simulink model "TESTENV_Task"  (R2020a)
settings: Solver=FixedStepAuto  StartTime=0.0  StopTime=4500  RelTol=1e-3
undefined symbols (not defined in the file or in its folder): airspeed1, ENUM_FlightTaskMode, ENUM_SensorHealthStatus, ENUM_SystemHealthStatus, FlightPerfParam_V10, FlightPerfParam_V1000, PlaneMode, radar1, SensorStatus, SystemHealthStatus, TaskParam_V10, TaskParam_V1000, windHeading_rad, windSpeed_ms
settings Model: PauseTimes=[500,868]  PacingRate=6  Creator=sl  LastModifiedBy=Administrator
settings DebuggingCC: InheritedTsInSrcMsg=none  ArithmeticOperatorsInVariantConditions=warning
settings ModelReferenceCC: PropagateVarSize=During execution
settings SFSimCC: CustomCodeUndefinedFunction=UseInterfaceOnly

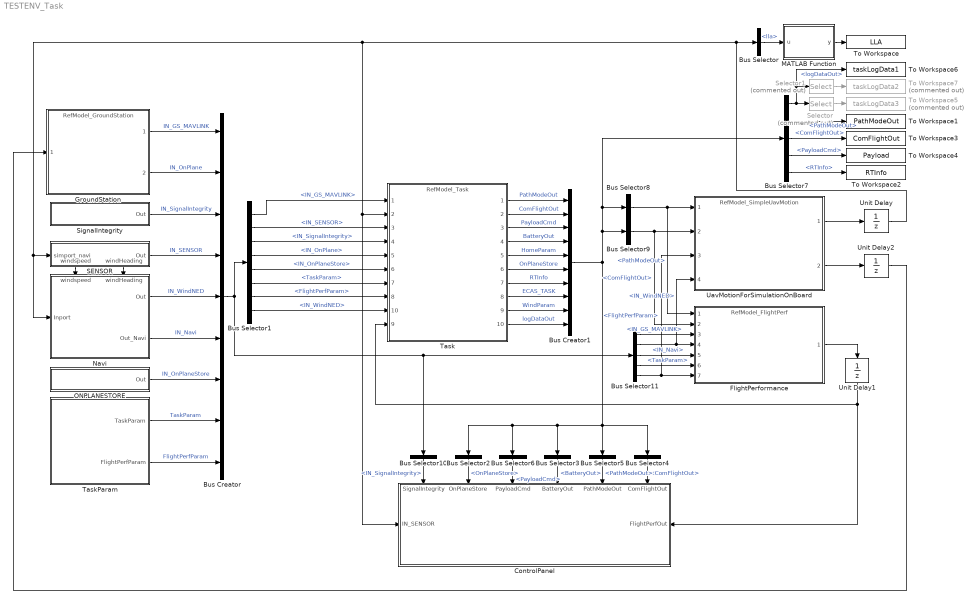
== system TESTENV_Task ==
  Bus Creator : BusCreator  Inputs=9
  Bus Creator1 : BusCreator  Inputs=10
  Bus Selector : BusSelector  OutputSignals=lla
  Bus Selector1 : BusSelector  OutputSignals=IN_GS_MAVLINK,IN_SENSOR,IN_SignalIntegrity,IN_OnPlane,IN_OnPlaneStore,TaskParam,FlightPerfParam,IN_WindNED
  Bus Selector10 : BusSelector  OutputSignals=IN_SignalIntegrity
  Bus Selector11 : BusSelector  OutputSignals=IN_GS_MAVLINK,IN_WindNED,IN_Navi,TaskParam,FlightPerfParam
  Bus Selector2 : BusSelector  OutputSignals=OnPlaneStore
  Bus Selector3 : BusSelector  OutputSignals=BatteryOut
  Bus Selector4 : BusSelector  OutputSignals=ComFlightOut
  Bus Selector5 : BusSelector  OutputSignals=PathModeOut
  Bus Selector6 : BusSelector  OutputSignals=PayloadCmd
  Bus Selector7 : BusSelector  OutputSignals=logDataOut,PathModeOut,ComFlightOut,PayloadCmd,RTInfo
  Bus Selector8 : BusSelector  OutputSignals=PathModeOut
  Bus Selector9 : BusSelector  OutputSignals=ComFlightOut
  ControlPanel : Subsystem
      settings: PortSchema="{\"entries\":[{\"content\":{\"sides\":[{\"content\":{\"connectorIds\":[]},\"type\":\"ConnectorPlacement.EquallySpacedRectSide\",\"uuid\":\"28eb3c17-6733-4c9d-9d3b-b06e91bad00c\"},{\"content\":{\"connectorIds\":[\"In3\",\"In4\",\"In5\",\"In6\",\"In7\",\"In8\"],\"side\":\"RIGHT\"},\"type\":\"ConnectorPlacement.EquallySpacedRectSide\",\"uuid\":\"44e37a17-9aaf-4985-a14b-a4ae4b690f0b\"},{\"content\":{\"connectorIds\":[\"In1\"],\"side\":\"TOP\"},\"type\":\"ConnectorPlacement.EquallySpacedRectSide\",\"uuid\":\"dc63a870-4d25-41e6-babc-24267acffaf6\"},{\"content\":{\"connectorIds\":[\"In2\"],\"side\":\"BOTTOM\"},\"type\":\"ConnectorPlacement.EquallySpacedRectSide\",\"uuid\":\"de4ecddf-9d24-4ca5-8235-aab9efd95b3c\"}]},\"type\":\"ConnectorPlacement.EquallySpacedConnector\",\"uuid\":\"a23d6a61-f1f8-4715-9225-859bb8c68d23\"}],\"packageUris\":[\"http://schema.mathworks.com/mf0/Connector/19700101\"],\"version\":\"1.0\"}"
  FlightPerformance : ModelReference  ModelNameDialog=RefModel_FlightPerf.slx  SimulationMode=Normal  CachedPortDiscreteRates=[0.04]  ModelReferenceVersion=1.3545
  GroundStation : ModelReference  ModelNameDialog=RefModel_GroundStation.slx  SimulationMode=Normal  CachedPortDiscreteRates=[0.04]  ModelReferenceVersion=1.3846
  MATLAB Function : MATLAB Function  TreatAsAtomicUnit=on
  Navi : Subsystem
      settings: PortSchema="{\"entries\":[{\"content\":{\"sides\":[{\"content\":{\"connectorIds\":[\"In1\"]},\"type\":\"ConnectorPlacement.EquallySpacedRectSide\",\"uuid\":\"f65589f5-bebe-42f0-87a0-22889f9d8cf8\"},{\"content\":{\"connectorIds\":[\"Out1\",\"Out2\"],\"side\":\"RIGHT\"},\"type\":\"ConnectorPlacement.EquallySpacedRectSide\",\"uuid\":\"9d118f62-a4fa-485f-8fb7-3972b29fb71e\"},{\"content\":{\"connectorIds\":[\"In2\",\"In3\"],\"side\":\"TOP\"},\"type\":\"ConnectorPlacement.EquallySpacedRectSide\",\"uuid\":\"31b3786a-ad94-4275-bb9f-8feeb00b35dc\"}]},\"type\":\"ConnectorPlacement.EquallySpacedConnector\",\"uuid\":\"aa2c1c65-c057-4fb8-aaff-4f4272248123\"}],\"packageUris\":[\"http://schema.mathworks.com/mf0/Connector/19700101\"],\"version\":\"1.0\"}"
  ONPLANESTORE : Subsystem
  SENSOR : Subsystem
      settings: PortSchema="{\"entries\":[{\"content\":{\"sides\":[{\"content\":{\"connectorIds\":[\"In1\"]},\"type\":\"ConnectorPlacement.EquallySpacedRectSide\",\"uuid\":\"ba991dc2-7a34-4bf6-a888-7f4af2e50d12\"},{\"content\":{\"connectorIds\":[\"Out1\"],\"side\":\"RIGHT\"},\"type\":\"ConnectorPlacement.EquallySpacedRectSide\",\"uuid\":\"c7226504-ba61-436f-baed-66203ae29e34\"},{\"content\":{\"connectorIds\":[],\"side\":\"TOP\"},\"type\":\"ConnectorPlacement.EquallySpacedRectSide\",\"uuid\":\"1861e618-12e2-4f65-bbab-d347bc046ba7\"},{\"content\":{\"connectorIds\":[\"Out2\",\"Out3\"],\"side\":\"BOTTOM\"},\"type\":\"ConnectorPlacement.EquallySpacedRectSide\",\"uuid\":\"711a3230-d97b-4007-957d-7ac810c9eb75\"}]},\"type\":\"ConnectorPlacement.EquallySpacedConnector\",\"uuid\":\"48c07c27-922c-4e4d-aad7-64a2a545d2e4\"}],\"packageUris\":[\"http://schema.mathworks.com/mf0/Connector/19700101\"],\"version\":\"1.0\"}"
  Selector : Selector  Commented=on  InputPortWidth=3  IndexOptions=Index vector (dialog)  Indices=3  OutputSizes=1
  Selector1 : Selector  Commented=on  InputPortWidth=3  IndexOptions=Index vector (dialog)  Indices=2  OutputSizes=1
  SignalIntegrity : Subsystem
  Task : ModelReference  ModelNameDialog=RefModel_Task.slx  SimulationMode=Normal  CachedPortDiscreteRates=[0.036]  ModelReferenceVersion=1.6002
      settings: PortSchema="{\"entries\":[{\"content\":{\"sides\":[{\"content\":{\"connectorIds\":[\"In1\",\"In2\",\"In3\",\"In4\",\"In5\",\"In6\",\"In7\",\"In8\",\"In10\",\"In9\"]},\"type\":\"ConnectorPlacement.EquallySpacedRectSide\",\"uuid\":\"d9fd24e3-43bd-49c5-a4e1-6245eb51949c\"},{\"content\":{\"connectorIds\":[\"Out1\",\"Out2\",\"Out3\",\"Out4\",\"Out5\",\"Out6\",\"Out7\",\"Out8\",\"Out9\",\"Out10\"],\"side\":\"RIGHT\"},\"type\":\"ConnectorPlacement.EquallySpacedRectSide\",\"uuid\":\"bf33909e-0e0f-4f0f-a250-56f1d45be6e7\"},{\"content\":{\"connectorIds\":[],\"side\":\"TOP\"},\"type\":\"ConnectorPlacement.EquallySpacedRectSide\",\"uuid\":\"77fc1f2c-3bac-4439-b1c1-53d076175420\"}]},\"type\":\"ConnectorPlacement.EquallySpacedConnector\",\"uuid\":\"17e9d58e-9274-43dc-be21-5439798aa13e\"}],\"packageUris\":[\"http://schema.mathworks.com/mf0/Connector/19700101\"],\"version\":\"1.0\"}"
  TaskParam : Subsystem
  To Workspace : ToWorkspace  VariableName=LLA  SaveFormat=Timeseries  SampleTime=-1
  To Workspace1 : ToWorkspace  VariableName=PathModeOut  SaveFormat=Timeseries  SampleTime=-1
  To Workspace2 : ToWorkspace  VariableName=RTInfo  SaveFormat=Timeseries  SampleTime=-1
  To Workspace3 : ToWorkspace  VariableName=ComFlightOut  SaveFormat=Timeseries  SampleTime=-1
  To Workspace4 : ToWorkspace  VariableName=Payload  SaveFormat=Timeseries  SampleTime=-1
  To Workspace5 : ToWorkspace  Commented=on  VariableName=taskLogData3  SaveFormat=Timeseries  SampleTime=-1
  To Workspace6 : ToWorkspace  VariableName=taskLogData1  SaveFormat=Timeseries  SampleTime=-1
  To Workspace7 : ToWorkspace  Commented=on  VariableName=taskLogData2  SaveFormat=Timeseries  SampleTime=-1
  UavMotionForSimulationOnBoard : ModelReference  ModelNameDialog=RefModel_SimpleUavMotion.slx  SimulationMode=Normal  CachedPortDiscreteRates=[0.04]  ModelReferenceVersion=1.1044
  Unit Delay : UnitDelay  SampleTime=-1  HasFrameUpgradeWarning=on
  Unit Delay1 : UnitDelay  SampleTime=-1  HasFrameUpgradeWarning=on
  Unit Delay2 : UnitDelay  SampleTime=-1  HasFrameUpgradeWarning=on
  wires:
  GroundStation/1 -> Bus Creator/1  "IN_GS_MAVLINK"
  SignalIntegrity/1(Out) -> Bus Creator/3  "IN_SignalIntegrity"
  GroundStation/2 -> Bus Creator/2  "IN_OnPlane"
  UavMotionForSimulationOnBoard/1 -> Unit Delay/1
  Unit Delay/1 -> ControlPanel/1(IN_SENSOR), Task/2, Navi/1(Inport), SENSOR/1(simport_navi), Bus Selector/1
  Bus Selector/1 -> MATLAB Function/1(u)  "<lla>"
  MATLAB Function/1(y) -> To Workspace/1
  SENSOR/1(Out) -> Bus Creator/4  "IN_SENSOR"
  ONPLANESTORE/1(Out) -> Bus Creator/7  "IN_OnPlaneStore"
  FlightPerformance/1 -> Unit Delay1/1
  Bus Selector1/6 -> Task/7  "<TaskParam>"
  Bus Creator/1 -> Bus Selector1/1, Bus Selector10/1, Bus Selector11/1
  Bus Selector1/1 -> Task/1  "<IN_GS_MAVLINK>"
  Bus Selector1/3 -> Task/4  "<IN_SignalIntegrity>"
  Bus Selector1/2 -> Task/3  "<IN_SENSOR>"
  Bus Selector1/4 -> Task/5  "<IN_OnPlane>"
  Bus Selector1/5 -> Task/6  "<IN_OnPlaneStore>"
  Task/1 -> Bus Creator1/1  "PathModeOut"
  Task/2 -> Bus Creator1/2  "ComFlightOut"
  Task/3 -> Bus Creator1/3  "PayloadCmd"
  Task/4 -> Bus Creator1/4  "BatteryOut"
  Task/5 -> Bus Creator1/5  "HomeParam"
  Task/6 -> Bus Creator1/6  "OnPlaneStore"
  Task/7 -> Bus Creator1/7  "RTInfo"
  Task/8 -> Bus Creator1/8  "ECAS_TASK"
  Task/9 -> Bus Creator1/9  "WindParam"
  Bus Selector2/1 -> ControlPanel/4(OnPlaneStore)  "<OnPlaneStore>"
  Bus Selector3/1 -> ControlPanel/6(BatteryOut)  "<BatteryOut>"
  Bus Selector4/1 -> ControlPanel/8(ComFlightOut)  "<ComFlightOut>"
  Bus Selector5/1 -> ControlPanel/7(PathModeOut)  "<PathModeOut>"
  Bus Selector6/1 -> ControlPanel/5(PayloadCmd)  "<PayloadCmd>"
  Bus Creator1/1 -> Bus Selector9/1, Bus Selector8/1, Bus Selector7/1, Bus Selector3/1, Bus Selector6/1, Bus Selector2/1, Bus Selector5/1, Bus Selector4/1
  Bus Selector7/5 -> To Workspace2/1  "<RTInfo>"
  Bus Selector7/2 -> To Workspace1/1  "<PathModeOut>"
  Bus Selector7/3 -> To Workspace3/1  "<ComFlightOut>"
  Bus Selector7/4 -> To Workspace4/1  "<PayloadCmd>"
  Bus Selector8/1 -> FlightPerformance/1, UavMotionForSimulationOnBoard/1  "<PathModeOut>"
  Bus Selector9/1 -> FlightPerformance/2, UavMotionForSimulationOnBoard/2  "<ComFlightOut>"
  Bus Selector10/1 -> ControlPanel/3(SignalIntegrity)  "<IN_SignalIntegrity>"
  Bus Selector11/1 -> FlightPerformance/3  "<IN_GS_MAVLINK>"
  Unit Delay1/1 -> Task/9, ControlPanel/2(FlightPerfOut)
  Navi/1(Out) -> Bus Creator/5  "IN_WindNED"
  SENSOR/2(windspeed) -> Navi/2(windspeed)
  Bus Selector1/8 -> Task/10  "<IN_WindNED>"
  Bus Selector11/2 -> FlightPerformance/4, UavMotionForSimulationOnBoard/4  "<IN_WindNED>"
  UavMotionForSimulationOnBoard/2 -> Unit Delay2/1
  Unit Delay2/1 -> GroundStation/1
  Task/10 -> Bus Creator1/10  "logDataOut"
  Bus Selector7/1 -> To Workspace6/1, Selector1/1, Selector/1  "<logDataOut>"
  Selector/1 -> To Workspace5/1
  Selector1/1 -> To Workspace7/1
  SENSOR/3(windHeading) -> Navi/3(windHeading)
  TaskParam/1(TaskParam) -> Bus Creator/8  "TaskParam"
  Navi/2(Out_Navi) -> Bus Creator/6  "IN_Navi"
  Bus Selector11/3 -> FlightPerformance/5  "<IN_Navi>"
  Bus Selector11/4 -> FlightPerformance/6  "<TaskParam>"
  TaskParam/2(FlightPerfParam) -> Bus Creator/9  "FlightPerfParam"
  Bus Selector1/7 -> Task/8  "<FlightPerfParam>"
  Bus Selector11/5 -> FlightPerformance/7, UavMotionForSimulationOnBoard/3  "<FlightPerfParam>"

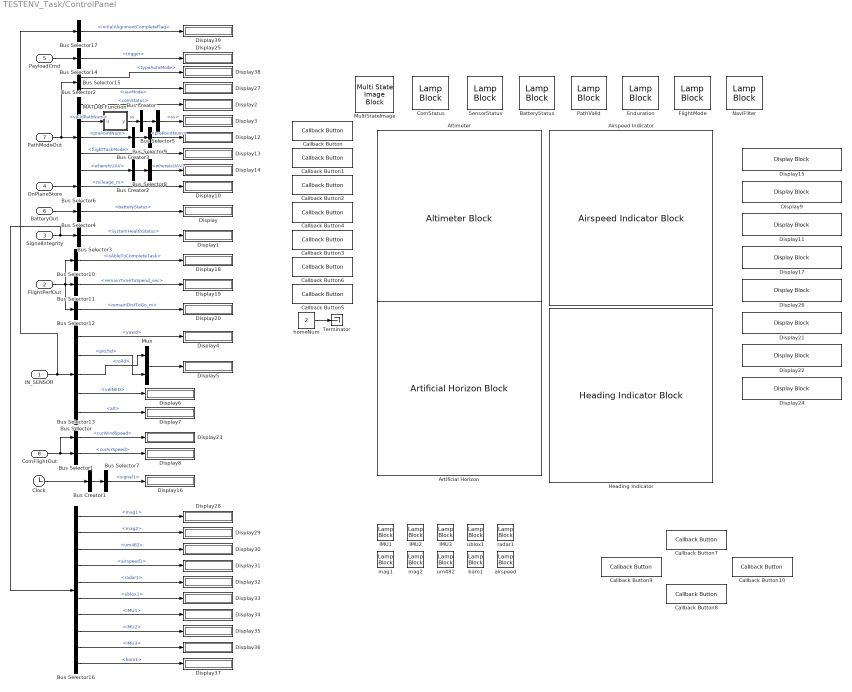
== system TESTENV_Task/ControlPanel ==
  IN_SENSOR : Inport
  FlightPerfOut : Inport  Port=2
  SignalIntegrity : Inport  Port=3
  OnPlaneStore : Inport  Port=4
  PayloadCmd : Inport  Port=5
  BatteryOut : Inport  Port=6
  PathModeOut : Inport  Port=7
  ComFlightOut : Inport  Port=8
  Airspeed Indicator : AirspeedIndicatorBlock  ScaleMin=-10  ScaleMax=50
  Altimeter : AltimeterBlock
  Artificial Horizon : ArtificialHorizonBlock
  BatteryStatus : LampBlock
  Bus Creator{,1..3} (4 alike) : BusCreator  Inputs=1
  Bus Selector : BusSelector  OutputSignals=yawd,pitchd,rolld,velNED,alt
  Bus Selector1 : BusSelector  OutputSignals=curAirSpeed
  Bus Selector10 : BusSelector  OutputSignals=isAbleToCompleteTask
  Bus Selector11 : BusSelector  OutputSignals=remainTimeToSpend_sec
  Bus Selector12 : BusSelector  OutputSignals=remainDistToGo_m
  Bus Selector13 : BusSelector  OutputSignals=curWindSpeed
  Bus Selector14 : BusSelector  OutputSignals=CAMERA.trigger
  Bus Selector15 : BusSelector  OutputSignals=typeAutoMode,uavMode
  Bus Selector16 : BusSelector  OutputSignals=SensorStatus.mag1,SensorStatus.mag2,SensorStatus.um482,SensorStatus.airspeed1,SensorStatus.radar1,SensorStatus.ublox1,SensorStatus.IMU1,SensorStatus.IMU2,SensorStatus.IMU3,SensorStatus.baro1
  Bus Selector17 : BusSelector  OutputSignals=initialAlignmentCompleteFlag
  Bus Selector2 : BusSelector  OutputSignals=comStatus,validPathNum,prePointNum,flightTaskMode,whereIsUAV
  Bus Selector3 : BusSelector  OutputSignals=SystemHealthStatus
  Bus Selector4 : BusSelector  OutputSignals=batteryStatus
  Bus Selector5 : BusSelector  OutputSignals=ss
  Bus Selector6 : BusSelector  OutputSignals=mileage_m
  Bus Selector7 : BusSelector  OutputSignals=signal1
  Bus Selector8 : BusSelector  OutputSignals=whereIsUAV
  Bus Selector9 : BusSelector  OutputSignals=prePointNum
  Callback Button : CallbackButton  ButtonText=起飞
      settings: ClickFcn=|
      | set_param('RefModel_GroundStation/GSButton','value','5')
      | tmpVal = get_param('RefModel_GroundStation/mav_command_long_recvflag','value');
      | tmpVal = str2double(tmpVal);
      | set_param('RefModel_GroundStation/mav_command_long_recvflag','value',num2str(tmpVal+1))
  Callback Button1 : CallbackButton  ButtonText=开始任务
      settings: ClickFcn=|
      | set_param('RefModel_GroundStation/GSButton','value','4')
      | tmpVal = get_param('RefModel_GroundStation/mav_command_long_recvflag','value');
      | tmpVal = str2double(tmpVal);
      | set_param('RefModel_GroundStation/mav_command_long_recvflag','value',num2str(tmpVal+1))
  Callback Button10 : CallbackButton  ButtonText=右+5
      settings: ClickFcn=|
      | tmpVal = get_param('RefModel_GroundStation/mavlink_msg_arrowkey/nRight','value');
      | tmpVal = str2double(tmpVal);
      | set_param('RefModel_GroundStation/mavlink_msg_arrowkey/nRight','value',num2str(tmpVal+5))
  Callback Button2 : CallbackButton  ButtonText=暂停
      settings: ClickFcn=|
      | set_param('RefModel_GroundStation/GSButton','value','3')
      | tmpVal = get_param('RefModel_GroundStation/mav_command_long_recvflag','value');
      | tmpVal = str2double(tmpVal);
      | set_param('RefModel_GroundStation/mav_command_long_recvflag','value',num2str(tmpVal+1))
  Callback Button3 : CallbackButton  ButtonText=返航
      settings: ClickFcn=|
      | set_param('RefModel_GroundStation/GSButton','value','2')
      | tmpVal = get_param('RefModel_GroundStation/mav_command_long_recvflag','value');
      | tmpVal = str2double(tmpVal);
      | set_param('RefModel_GroundStation/mav_command_long_recvflag','value',num2str(tmpVal+1))
  Callback Button4 : CallbackButton  ButtonText=固定翼转旋翼
      settings: ClickFcn=|
      | set_param('RefModel_GroundStation/GSButton','value','14')
      | tmpVal = get_param('RefModel_GroundStation/mav_command_long_recvflag','value');
      | tmpVal = str2double(tmpVal);
      | set_param('RefModel_GroundStation/mav_command_long_recvflag','value',num2str(tmpVal+1))
  Callback Button5 : CallbackButton  ButtonText=修改HOME点
      settings: ClickFcn=|
      | tmpVal = get_param('TESTENV_Task/ControlPanel/homeNum','value');
      | tmpVal = str2double(tmpVal);
      | if tmpVal > 4
      |     tmpVal = 4;
      | elseif tmpVal < 1
      |     tmpVal = 1;
      | end
      | set_param('RefModel_GroundStation/PathPoints/HomeNumSel','value',num2str(tmpVal))
  Callback Button6 : CallbackButton  ButtonText=一键降落
      settings: ClickFcn=|
      | set_param('RefModel_GroundStation/GSButton','value','7')
      | tmpVal = get_param('RefModel_GroundStation/mav_command_long_recvflag','value');
      | tmpVal = str2double(tmpVal);
      | set_param('RefModel_GroundStation/mav_command_long_recvflag','value',num2str(tmpVal+1))
  Callback Button7 : CallbackButton  ButtonText=前+5
      settings: ClickFcn=|
      | tmpVal = get_param('RefModel_GroundStation/mavlink_msg_arrowkey/nFront','value');
      | tmpVal = str2double(tmpVal);
      | set_param('RefModel_GroundStation/mavlink_msg_arrowkey/nFront','value',num2str(tmpVal+5))
  Callback Button8 : CallbackButton  ButtonText=后+5
      settings: ClickFcn=|
      | tmpVal = get_param('RefModel_GroundStation/mavlink_msg_arrowkey/nBack','value');
      | tmpVal = str2double(tmpVal);
      | set_param('RefModel_GroundStation/mavlink_msg_arrowkey/nBack','value',num2str(tmpVal+5))
  Callback Button9 : CallbackButton  ButtonText=左+5
      settings: ClickFcn=|
      | tmpVal = get_param('RefModel_GroundStation/mavlink_msg_arrowkey/nLeft','value');
      | tmpVal = str2double(tmpVal);
      | set_param('RefModel_GroundStation/mavlink_msg_arrowkey/nLeft','value',num2str(tmpVal+5))
  Clock : Clock
  ComStatus : LampBlock
  Display{,1..8,10,12..14,16,18..20,23,25,27..39} (32 alike) : Display
  Display11 : DisplayBlock  Format=Custom  Transparency=1  FormatString=时间 %.1f [sec]
  Display15 : DisplayBlock  Format=Custom  Transparency=1  FormatString=%s
  Display17 : DisplayBlock  Format=Custom  Transparency=1  FormatString=航点 %d
  Display21 : DisplayBlock  Format=Custom  Transparency=1  FormatString=剩余时间 %.0f [s]
  Display22 : DisplayBlock  Format=Custom  Transparency=1  FormatString=剩余航程 %.0f [m]
  Display24 : DisplayBlock  Format=Custom  Transparency=1  FormatString=风速 %.1f [m/s]
  Display26 : DisplayBlock  Format=Custom  Transparency=1  FormatString=拍照点 %.0f
  Display9 : DisplayBlock  Format=Custom  Transparency=1  FormatString=里程 %.0f [m]
  Enduration : LampBlock
  FlightMode : LampBlock
  Heading Indicator : HeadingIndicatorBlock
  IMU1 : LampBlock
  IMU2 : LampBlock
  IMU3 : LampBlock
  MATLAB Function : MATLAB Function  TreatAsAtomicUnit=on
  MultiStateImage : MultiStateImageBlock
  Mux : Mux  Inputs=2
  NaviFilter : LampBlock
  PathValid : LampBlock
  SensorStatus : LampBlock
  Terminator : Terminator
  airspeed : LampBlock
  baro1 : LampBlock
  homeNum : Constant  Value=2
  mag1 : LampBlock
  mag2 : LampBlock
  radar1 : LampBlock
  ublox1 : LampBlock
  um482 : LampBlock
  wires:
  Bus Selector/1 -> Display4/1  "<yawd>"
  Bus Selector/4 -> Display6/1  "<velNED>"
  Bus Selector/5 -> Display7/1  "<alt>"
  ComFlightOut/1 -> Bus Selector13/1, Bus Selector1/1
  Bus Selector1/1 -> Display8/1  "<curAirSpeed>"
  Mux/1 -> Display5/1
  Bus Selector/2 -> Mux/2  "<pitchd>"
  Bus Selector/3 -> Mux/1  "<rolld>"
  PathModeOut/1 -> Bus Selector15/1, Bus Selector2/1
  Bus Selector2/1 -> Display2/1  "<comStatus>"
  SignalIntegrity/1 -> Bus Selector16/1, Bus Selector3/1
  Bus Selector3/1 -> Display1/1  "<SystemHealthStatus>"
  BatteryOut/1 -> Bus Selector4/1
  Bus Selector4/1 -> Display/1  "<batteryStatus>"
  Bus Selector2/2 -> MATLAB Function/1(u)  "<validPathNum>"
  MATLAB Function/1(y) -> Bus Creator/1  "ss"
  Bus Selector5/1 -> Display3/1  "<ss>"
  Bus Creator/1 -> Bus Selector5/1
  OnPlaneStore/1 -> Bus Selector6/1
  Bus Selector6/1 -> Display10/1  "<mileage_m>"
  Bus Selector2/4 -> Display13/1  "<flightTaskMode>"
  Bus Creator1/1 -> Bus Selector7/1
  Bus Selector7/1 -> Display16/1  "<signal1>"
  Clock/1 -> Bus Creator1/1
  Bus Creator2/1 -> Bus Selector8/1
  Bus Selector2/5 -> Bus Creator2/1  "<whereIsUAV>"
  Bus Selector8/1 -> Display14/1  "<whereIsUAV>"
  Bus Creator3/1 -> Bus Selector9/1
  Bus Selector9/1 -> Display12/1  "<prePointNum>"
  Bus Selector2/3 -> Bus Creator3/1  "<prePointNum>"
  FlightPerfOut/1 -> Bus Selector10/1, Bus Selector12/1, Bus Selector11/1
  Bus Selector10/1 -> Display18/1  "<isAbleToCompleteTask>"
  Bus Selector11/1 -> Display19/1  "<remainTimeToSpend_sec>"
  Bus Selector12/1 -> Display20/1  "<remainDistToGo_m>"
  Bus Selector13/1 -> Display23/1  "<curWindSpeed>"
  Bus Selector14/1 -> Display25/1  "<trigger>"
  PayloadCmd/1 -> Bus Selector14/1
  Bus Selector15/2 -> Display27/1  "<uavMode>"
  Bus Selector16/1 -> Display28/1  "<mag1>"
  Bus Selector16/2 -> Display29/1  "<mag2>"
  Bus Selector16/3 -> Display30/1  "<um482>"
  Bus Selector16/4 -> Display31/1  "<airspeed1>"
  Bus Selector16/5 -> Display32/1  "<radar1>"
  Bus Selector16/6 -> Display33/1  "<ublox1>"
  Bus Selector16/7 -> Display34/1  "<IMU1>"
  Bus Selector16/8 -> Display35/1  "<IMU2>"
  Bus Selector16/9 -> Display36/1  "<IMU3>"
  Bus Selector16/10 -> Display37/1  "<baro1>"
  Bus Selector15/1 -> Display38/1  "<typeAutoMode>"
  IN_SENSOR/1 -> Bus Selector17/1, Bus Selector/1
  Bus Selector17/1 -> Display39/1  "<initialAlignmentCompleteFlag>"
  homeNum/1 -> Terminator/1

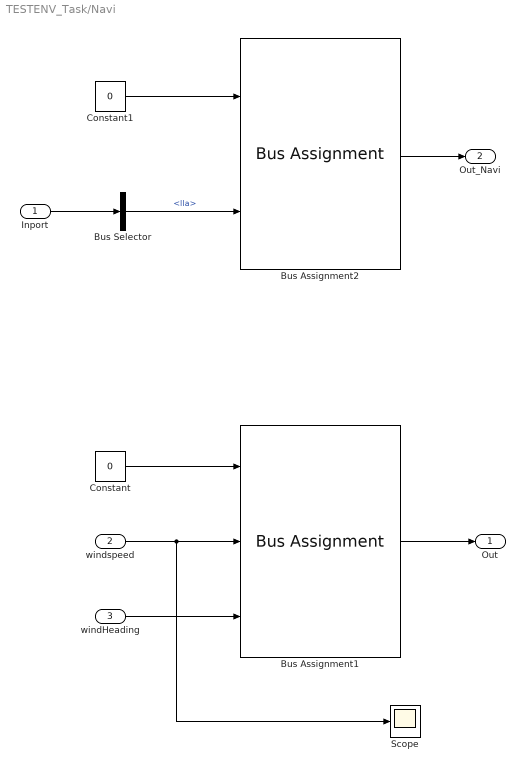
== system TESTENV_Task/Navi ==
  Inport : Inport
  windspeed : Inport  Port=2
  windHeading : Inport  Port=3
  Bus Assignment1 : BusAssignment  AssignedSignals=windSpeed_ms,windHeading_rad
  Bus Assignment2 : BusAssignment  AssignedSignals=lla
  Bus Selector : BusSelector  OutputSignals=lla
  Constant : Constant  Value=0  OutDataTypeStr=Bus: BUS_NAVI_GlobalWindEst
  Constant1 : Constant  Value=0  OutDataTypeStr=Bus: BUS_NAVI_TO_FIRM
  Scope : Scope
  Out : Outport
  Out_Navi : Outport  Port=2  BusOutputAsStruct=on
  wires:
  Bus Assignment1/1 -> Out/1
  Constant/1 -> Bus Assignment1/1
  windspeed/1 -> Scope/1, Bus Assignment1/2
  windHeading/1 -> Bus Assignment1/3
  Constant1/1 -> Bus Assignment2/1
  Bus Assignment2/1 -> Out_Navi/1
  Inport/1 -> Bus Selector/1
  Bus Selector/1 -> Bus Assignment2/2  "<lla>"

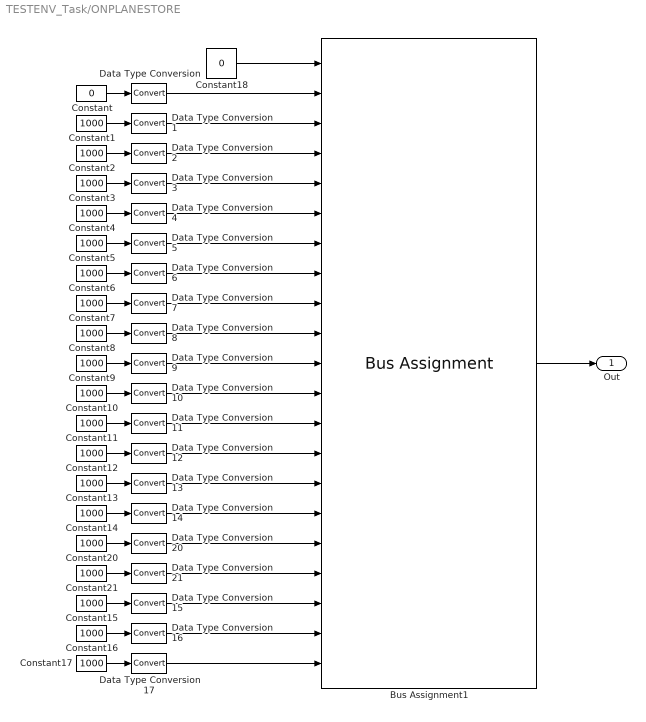
== system TESTENV_Task/ONPLANESTORE ==
  Bus Assignment1 : BusAssignment  AssignedSignals=isDataValid,mileage_m,Number.sortie,Number.nTakeOff,Number.nPowerOn,Number.nPath,Number.nLand,Number.nRotor2Fix,Number.nFix2Rotor,Duration.fixInAir,Duration.rotorInAir,Duration.rotorOnGround,Duration.fixAirSpeed_0_10,Duration.fixAirSpeed_10_20,Duration.fixAirSpeed_20_30,Duration.fixAirSpeed_30_40,Duration.rotorSpeed_0_5,Duration.rotorSpeed_5_10,Duration.rotorSpeed_10_20,Duration.rotorSpeed_20_30
  Constant : Constant  Value=0
  Constant{1..17,20..21} (19 alike) : Constant  Value=1000
  Constant18 : Constant  Value=0  OutDataTypeStr=Bus: BUS_ONPLANE_STORE
  Data Type Conversion{,1..17,20..21} (20 alike) : DataTypeConversion
  Out : Outport
  wires:
  Bus Assignment1/1 -> Out/1
  Data Type Conversion/1 -> Bus Assignment1/2
  Constant18/1 -> Bus Assignment1/1
  Constant/1 -> Data Type Conversion/1
  Constant1/1 -> Data Type Conversion1/1
  Data Type Conversion1/1 -> Bus Assignment1/3
  Constant3/1 -> Data Type Conversion3/1
  Constant2/1 -> Data Type Conversion2/1
  Data Type Conversion3/1 -> Bus Assignment1/5
  Data Type Conversion2/1 -> Bus Assignment1/4
  Data Type Conversion6/1 -> Bus Assignment1/8
  Data Type Conversion7/1 -> Bus Assignment1/9
  Constant6/1 -> Data Type Conversion6/1
  Constant7/1 -> Data Type Conversion7/1
  Data Type Conversion5/1 -> Bus Assignment1/7
  Constant5/1 -> Data Type Conversion5/1
  Constant4/1 -> Data Type Conversion4/1
  Data Type Conversion4/1 -> Bus Assignment1/6
  Data Type Conversion11/1 -> Bus Assignment1/13
  Constant11/1 -> Data Type Conversion11/1
  Constant12/1 -> Data Type Conversion12/1
  Data Type Conversion12/1 -> Bus Assignment1/14
  Constant14/1 -> Data Type Conversion14/1
  Constant13/1 -> Data Type Conversion13/1
  Data Type Conversion14/1 -> Bus Assignment1/16
  Data Type Conversion13/1 -> Bus Assignment1/15
  Data Type Conversion9/1 -> Bus Assignment1/11
  Data Type Conversion10/1 -> Bus Assignment1/12
  Constant9/1 -> Data Type Conversion9/1
  Constant10/1 -> Data Type Conversion10/1
  Data Type Conversion8/1 -> Bus Assignment1/10
  Constant8/1 -> Data Type Conversion8/1
  Constant20/1 -> Data Type Conversion20/1
  Constant15/1 -> Data Type Conversion15/1
  Constant21/1 -> Data Type Conversion21/1
  Constant17/1 -> Data Type Conversion17/1
  Constant16/1 -> Data Type Conversion16/1
  Data Type Conversion20/1 -> Bus Assignment1/17
  Data Type Conversion21/1 -> Bus Assignment1/18
  Data Type Conversion15/1 -> Bus Assignment1/19
  Data Type Conversion16/1 -> Bus Assignment1/20
  Data Type Conversion17/1 -> Bus Assignment1/21

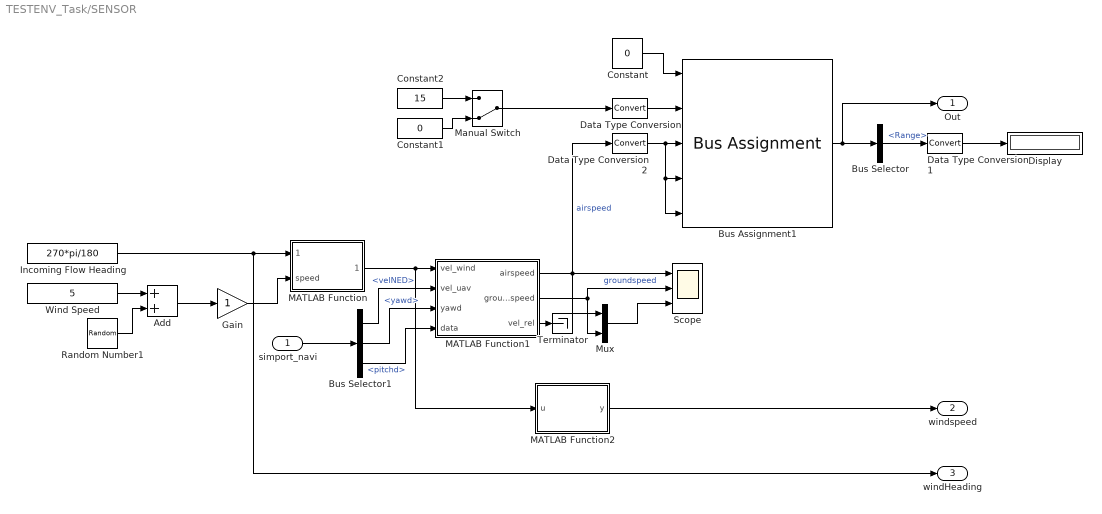
== system TESTENV_Task/SENSOR ==
  simport_navi : Inport
  Add : Sum
  Bus Assignment1 : BusAssignment  AssignedSignals=radar1.Range,airspeed1.airspeed,airspeed1.airspeed_true,airspeed1.airspeed_indicate
  Bus Selector : BusSelector  OutputSignals=radar1.Range
  Bus Selector1 : BusSelector  OutputSignals=velNED,yawd,pitchd
  Constant : Constant  Value=0  OutDataTypeStr=Bus: BUS_SENSOR
  Constant1 : Constant  Value=0
  Constant2 : Constant  Value=15
  Data Type Conversion : DataTypeConversion
  Data Type Conversion1 : DataTypeConversion
  Data Type Conversion2 : DataTypeConversion
  Display : Display
  Gain : Gain
  Incoming Flow Heading : Constant  Value=270*pi/180
  MATLAB Function : MATLAB Function  TreatAsAtomicUnit=on
  MATLAB Function1 : MATLAB Function  TreatAsAtomicUnit=on
  MATLAB Function2 : MATLAB Function  TreatAsAtomicUnit=on
  Manual Switch : ManualSwitch  CurrentSetting=0
  Mux : Mux  Inputs=2
  Random Number1 : RandomNumber  Variance=0.5^2  Seed=123
  Scope : Scope  NumInputPorts=3
  Terminator : Terminator
  Wind Speed : Constant  Value=5
  Out : Outport
  windspeed : Outport  Port=2
  windHeading : Outport  Port=3
  wires:
  Bus Selector/1 -> Data Type Conversion1/1  "<Range>"
  Constant2/1 -> Manual Switch/1
  Constant/1 -> Bus Assignment1/1
  Manual Switch/1 -> Data Type Conversion/1
  Constant1/1 -> Manual Switch/2
  Data Type Conversion/1 -> Bus Assignment1/2
  Bus Assignment1/1 -> Out/1, Bus Selector/1
  Data Type Conversion1/1 -> Display/1
  Incoming Flow Heading/1 -> windHeading/1, MATLAB Function/1(heading)
  simport_navi/1 -> Bus Selector1/1
  MATLAB Function/1(velNED_wind) -> MATLAB Function2/1(u), MATLAB Function1/1(vel_wind)
  Bus Selector1/1 -> MATLAB Function1/2(vel_uav)  "<velNED>"
  MATLAB Function1/2(groundspeed) -> Scope/2, Mux/2  "groundspeed"
  Mux/1 -> Scope/3
  MATLAB Function1/1(airspeed) -> Data Type Conversion2/1, Scope/1, Mux/1  "airspeed"
  Bus Selector1/2 -> MATLAB Function1/3(yawd)  "<yawd>"
  Bus Selector1/3 -> MATLAB Function1/4(data)  "<pitchd>"
  Wind Speed/1 -> Add/1
  Random Number1/1 -> Add/2
  Add/1 -> Gain/1
  Gain/1 -> MATLAB Function/2(speed)
  MATLAB Function2/1(y) -> windspeed/1
  Data Type Conversion2/1 -> Bus Assignment1/4, Bus Assignment1/5, Bus Assignment1/3
  MATLAB Function1/3(vel_rel) -> Terminator/1

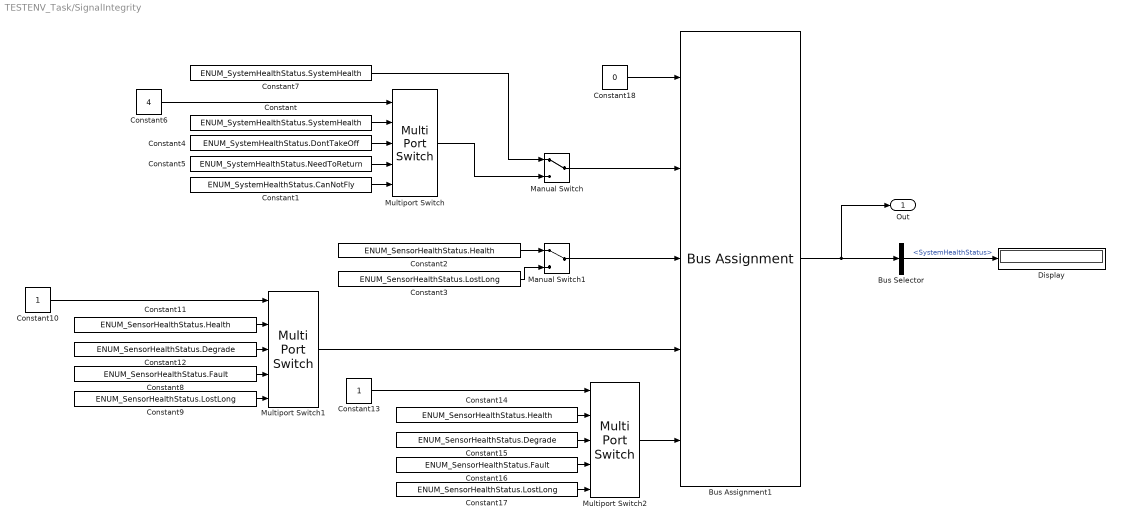
== system TESTENV_Task/SignalIntegrity ==
  Bus Assignment1 : BusAssignment  AssignedSignals=SystemHealthStatus,SensorStatus.radar1,SensorStatus.ublox1,SensorStatus.um482
  Bus Selector : BusSelector  OutputSignals=SystemHealthStatus
  Constant : Constant  Value=ENUM_SystemHealthStatus.SystemHealth  OutDataTypeStr=Enum: ENUM_SystemHealthStatus
  Constant1 : Constant  Value=ENUM_SystemHealthStatus.CanNotFly  OutDataTypeStr=Enum: ENUM_SystemHealthStatus
  Constant10 : Constant
  Constant11 : Constant  Value=ENUM_SensorHealthStatus.Health  OutDataTypeStr=Enum: ENUM_SensorHealthStatus
  Constant12 : Constant  Value=ENUM_SensorHealthStatus.Degrade  OutDataTypeStr=Enum: ENUM_SensorHealthStatus
  Constant13 : Constant
  Constant14 : Constant  Value=ENUM_SensorHealthStatus.Health  OutDataTypeStr=Enum: ENUM_SensorHealthStatus
  Constant15 : Constant  Value=ENUM_SensorHealthStatus.Degrade  OutDataTypeStr=Enum: ENUM_SensorHealthStatus
  Constant16 : Constant  Value=ENUM_SensorHealthStatus.Fault  OutDataTypeStr=Enum: ENUM_SensorHealthStatus
  Constant17 : Constant  Value=ENUM_SensorHealthStatus.LostLong  OutDataTypeStr=Enum: ENUM_SensorHealthStatus
  Constant18 : Constant  Value=0  OutDataTypeStr=Bus: BUS_NAVI_SensorSignalIntegrity
  Constant2 : Constant  Value=ENUM_SensorHealthStatus.Health  OutDataTypeStr=Enum: ENUM_SensorHealthStatus
  Constant3 : Constant  Value=ENUM_SensorHealthStatus.LostLong  OutDataTypeStr=Enum: ENUM_SensorHealthStatus
  Constant4 : Constant  Value=ENUM_SystemHealthStatus.DontTakeOff  OutDataTypeStr=Enum: ENUM_SystemHealthStatus
  Constant5 : Constant  Value=ENUM_SystemHealthStatus.NeedToReturn  OutDataTypeStr=Enum: ENUM_SystemHealthStatus
  Constant6 : Constant  Value=4
  Constant7 : Constant  Value=ENUM_SystemHealthStatus.SystemHealth  OutDataTypeStr=Enum: ENUM_SystemHealthStatus
  Constant8 : Constant  Value=ENUM_SensorHealthStatus.Fault  OutDataTypeStr=Enum: ENUM_SensorHealthStatus
  Constant9 : Constant  Value=ENUM_SensorHealthStatus.LostLong  OutDataTypeStr=Enum: ENUM_SensorHealthStatus
  Display : Display
  Manual Switch : ManualSwitch
  Manual Switch1 : ManualSwitch
  Multiport Switch : MultiPortSwitch  Inputs=4
  Multiport Switch1 : MultiPortSwitch  Inputs=4
  Multiport Switch2 : MultiPortSwitch  Inputs=4
  Out : Outport
  wires:
  Manual Switch/1 -> Bus Assignment1/2
  Constant18/1 -> Bus Assignment1/1
  Constant7/1 -> Manual Switch/1
  Multiport Switch/1 -> Manual Switch/2
  Bus Assignment1/1 -> Out/1, Bus Selector/1
  Bus Selector/1 -> Display/1  "<SystemHealthStatus>"
  Constant3/1 -> Manual Switch1/2
  Constant2/1 -> Manual Switch1/1
  Manual Switch1/1 -> Bus Assignment1/3
  Constant/1 -> Multiport Switch/2
  Constant4/1 -> Multiport Switch/3
  Constant5/1 -> Multiport Switch/4
  Constant1/1 -> Multiport Switch/5
  Constant6/1 -> Multiport Switch/1
  Constant10/1 -> Multiport Switch1/1
  Constant12/1 -> Multiport Switch1/3
  Constant11/1 -> Multiport Switch1/2
  Constant8/1 -> Multiport Switch1/4
  Constant9/1 -> Multiport Switch1/5
  Multiport Switch1/1 -> Bus Assignment1/4
  Constant15/1 -> Multiport Switch2/3
  Constant17/1 -> Multiport Switch2/5
  Constant16/1 -> Multiport Switch2/4
  Constant13/1 -> Multiport Switch2/1
  Constant14/1 -> Multiport Switch2/2
  Multiport Switch2/1 -> Bus Assignment1/5

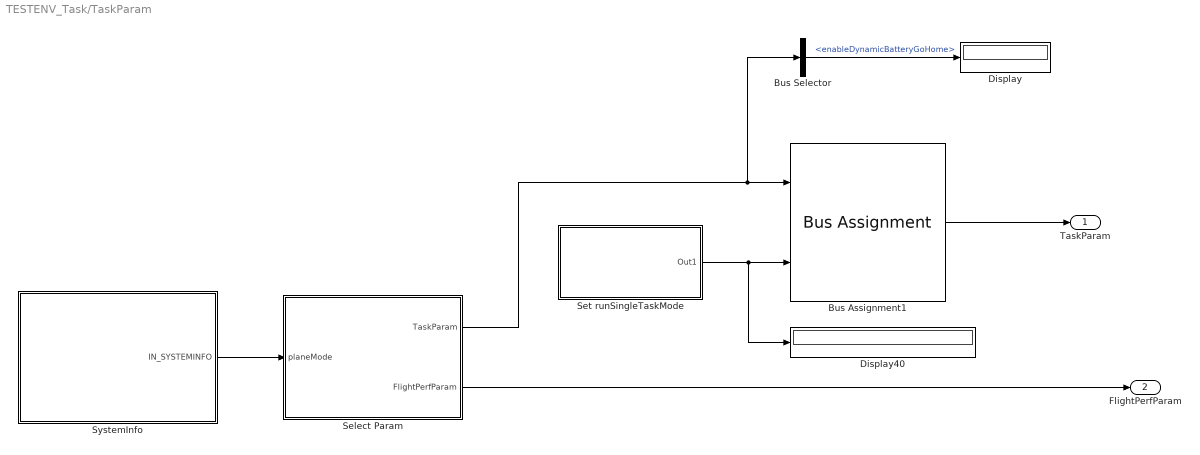
== system TESTENV_Task/TaskParam ==
  Bus Assignment1 : BusAssignment  AssignedSignals=runSingleTaskMode
  Bus Selector : BusSelector  OutputSignals=enableDynamicBatteryGoHome
  Display : Display
  Display40 : Display
  Select Param : Subsystem
  Set runSingleTaskMode : Subsystem
  SystemInfo : Subsystem
  TaskParam : Outport
  FlightPerfParam : Outport  Port=2
  wires:
  Select Param/1(TaskParam) -> Bus Selector/1, Bus Assignment1/1
  Bus Assignment1/1 -> TaskParam/1
  Set runSingleTaskMode/1(Out1) -> Display40/1, Bus Assignment1/2
  Select Param/2(FlightPerfParam) -> FlightPerfParam/1
  SystemInfo/1(IN_SYSTEMINFO) -> Select Param/1(planeMode)
  Bus Selector/1 -> Display/1  "<enableDynamicBatteryGoHome>"

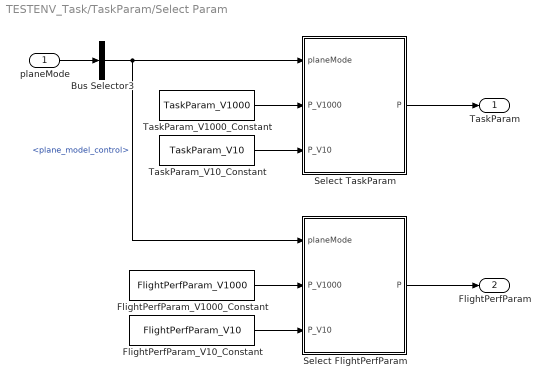
== system TESTENV_Task/TaskParam/Select Param ==
  planeMode : Inport
  Bus Selector3 : BusSelector  OutputSignals=plane_model_control
  FlightPerfParam_V1000_Constant : Constant  Value=FlightPerfParam_V1000  OutDataTypeStr=Bus: BUS_FLIGHTPERF_PARAM
  FlightPerfParam_V10_Constant : Constant  Value=FlightPerfParam_V10  OutDataTypeStr=Bus: BUS_FLIGHTPERF_PARAM
  Select FlightPerfParam : MATLAB Function  TreatAsAtomicUnit=on
  Select TaskParam : MATLAB Function  TreatAsAtomicUnit=on
  TaskParam_V1000_Constant : Constant  Value=TaskParam_V1000  OutDataTypeStr=Bus: BUS_TASK_PATH_AlgoParam
  TaskParam_V10_Constant : Constant  Value=TaskParam_V10  OutDataTypeStr=Bus: BUS_TASK_PATH_AlgoParam
  TaskParam : Outport
  FlightPerfParam : Outport  Port=2
  wires:
  TaskParam_V1000_Constant/1 -> Select TaskParam/2(P_V1000)
  TaskParam_V10_Constant/1 -> Select TaskParam/3(P_V10)
  Select TaskParam/1(P) -> TaskParam/1
  planeMode/1 -> Bus Selector3/1
  Bus Selector3/1 -> Select FlightPerfParam/1(planeMode), Select TaskParam/1(planeMode)  "<plane_model_control>"
  FlightPerfParam_V10_Constant/1 -> Select FlightPerfParam/3(P_V10)
  FlightPerfParam_V1000_Constant/1 -> Select FlightPerfParam/2(P_V1000)
  Select FlightPerfParam/1(P) -> FlightPerfParam/1

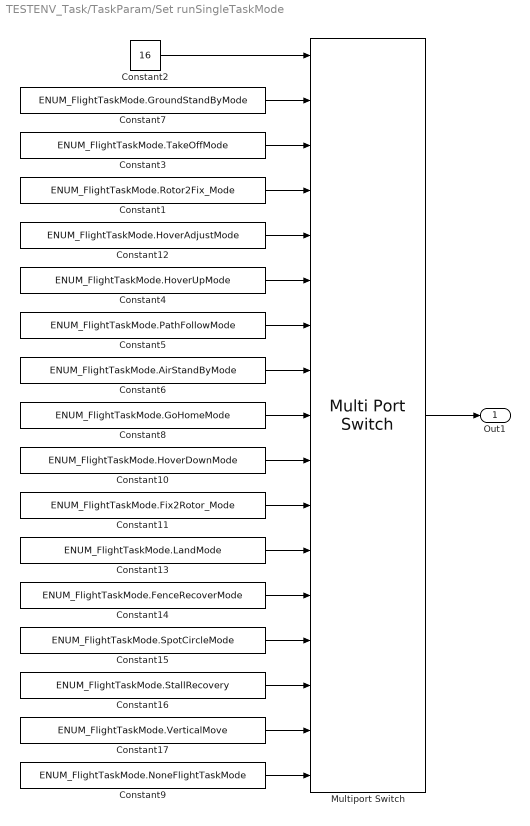
== system TESTENV_Task/TaskParam/Set runSingleTaskMode ==
  Constant1 : Constant  Value=ENUM_FlightTaskMode.Rotor2Fix_Mode
  Constant10 : Constant  Value=ENUM_FlightTaskMode.HoverDownMode
  Constant11 : Constant  Value=ENUM_FlightTaskMode.Fix2Rotor_Mode
  Constant12 : Constant  Value=ENUM_FlightTaskMode.HoverAdjustMode
  Constant13 : Constant  Value=ENUM_FlightTaskMode.LandMode
  Constant14 : Constant  Value=ENUM_FlightTaskMode.FenceRecoverMode
  Constant15 : Constant  Value=ENUM_FlightTaskMode.SpotCircleMode
  Constant16 : Constant  Value=ENUM_FlightTaskMode.StallRecovery
  Constant17 : Constant  Value=ENUM_FlightTaskMode.VerticalMove
  Constant2 : Constant  Value=16
  Constant3 : Constant  Value=ENUM_FlightTaskMode.TakeOffMode
  Constant4 : Constant  Value=ENUM_FlightTaskMode.HoverUpMode
  Constant5 : Constant  Value=ENUM_FlightTaskMode.PathFollowMode
  Constant6 : Constant  Value=ENUM_FlightTaskMode.AirStandByMode
  Constant7 : Constant  Value=ENUM_FlightTaskMode.GroundStandByMode
  Constant8 : Constant  Value=ENUM_FlightTaskMode.GoHomeMode
  Constant9 : Constant  Value=ENUM_FlightTaskMode.NoneFlightTaskMode
  Multiport Switch : MultiPortSwitch  Inputs=16  DiagnosticForDefault=Warning
  Out1 : Outport
  wires:
  Constant12/1 -> Multiport Switch/5
  Constant11/1 -> Multiport Switch/11
  Constant6/1 -> Multiport Switch/8
  Constant3/1 -> Multiport Switch/3
  Constant15/1 -> Multiport Switch/14
  Constant16/1 -> Multiport Switch/15
  Constant7/1 -> Multiport Switch/2
  Constant9/1 -> Multiport Switch/17
  Constant4/1 -> Multiport Switch/6
  Constant13/1 -> Multiport Switch/12
  Constant1/1 -> Multiport Switch/4
  Constant14/1 -> Multiport Switch/13
  Constant8/1 -> Multiport Switch/9
  Constant5/1 -> Multiport Switch/7
  Constant17/1 -> Multiport Switch/16
  Constant2/1 -> Multiport Switch/1
  Constant10/1 -> Multiport Switch/10
  Multiport Switch/1 -> Out1/1

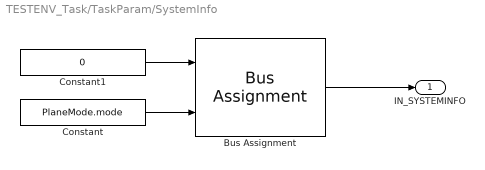
== system TESTENV_Task/TaskParam/SystemInfo ==
  Bus Assignment : BusAssignment  AssignedSignals=plane_model_control
  Constant : Constant  Value=PlaneMode.mode  OutDataTypeStr=Enum: ENUM_plane_mode
  Constant1 : Constant  Value=0  OutDataTypeStr=Bus: BUS_SYSTEMINFO_INPUT
  IN_SYSTEMINFO : Outport
  wires:
  Constant1/1 -> Bus Assignment/1
  Constant/1 -> Bus Assignment/2
  Bus Assignment/1 -> IN_SYSTEMINFO/1

== matlab function TESTENV_Task/SENSOR/MATLAB Function ==
  data: heading input; velNED_wind output; speed input
function velNED_wind = fcn(heading,speed)
persistent pSpeed
if isempty(pSpeed)
    pSpeed = speed;
end
k = 0.8;
pSpeed = k*pSpeed + (1-k)*speed;
velNED_wind = pSpeed*[cos(heading);sin(heading);0];

== matlab function TESTENV_Task/MATLAB Function ==
  data: u input; y output
function y = fcn(u)
if u(1) == 0
    y = nan*u;
else
    y = u;
end

== matlab function TESTENV_Task/SENSOR/MATLAB Function1 ==
  data: vel_wind input; airspeed output; groundspeed output; vel_uav input; vel_rel output; yawd input; data input
function [airspeed,groundspeed,vel_rel] = fcn(vel_wind,vel_uav, yawd, data)
vel_rel = vel_wind + vel_uav;
airspeedNorm = norm(vel_rel(1:2));
windInc = atan2(vel_wind(2),vel_wind(1));
dyaw = angdiff(yawd*pi/180,windInc);
windvel_alongheading = cos(dyaw)*norm(vel_wind(1:2));
airspeed = norm(vel_uav(1:2)) + windvel_alongheading;
% airspeed = airspeedNorm;
groundspeed = norm(vel_uav(1:2));
% fprintf('airspeed:%.0f,airspeed1:%.0f\n',airspeed,airspeed1)

== matlab function TESTENV_Task/ControlPanel/MATLAB Function ==
  data: u input; y output
function y = fcn(u)
if u > 0
    y = true;
else
    y = false;
end

== matlab function TESTENV_Task/SENSOR/MATLAB Function2 ==
  data: u input; y output
function y = fcn(u)
y = norm(u);

== matlab function TESTENV_Task/TaskParam/Select Param/Select TaskParam ==
  data: planeMode input Enum: ENUM_plane_mode; P output Bus: BUS_TASK_PATH_AlgoParam; P_V1000 input Bus: BUS_TASK_PATH_AlgoParam; P_V10 input Bus: BUS_TASK_PATH_AlgoParam
function P = fcn(planeMode,P_V1000,P_V10)
switch planeMode
    case ENUM_plane_mode.V10
        P = P_V10;
    case {ENUM_plane_mode.V1000,ENUM_plane_mode.V10s}
        P = P_V1000;
    otherwise
        P = P_V1000;
end

== matlab function TESTENV_Task/TaskParam/Select Param/Select FlightPerfParam ==
  data: planeMode input Enum: ENUM_plane_mode; P output Bus: BUS_FLIGHTPERF_PARAM; P_V1000 input Bus: BUS_FLIGHTPERF_PARAM; P_V10 input Bus: BUS_FLIGHTPERF_PARAM
function P = fcn(planeMode,P_V1000,P_V10)
switch planeMode
    case ENUM_plane_mode.V10
        P = P_V10;
    case {ENUM_plane_mode.V1000,ENUM_plane_mode.V10s}
        P = P_V1000;
    otherwise
        P = P_V1000;
end
